simulink model "stepMotor"  (R2023b)
settings: Solver=FixedStepDiscrete  StartTime=0.0  StopTime=0.5  FixedStep=0.0001  RelTol=1e-3  EnableMultiTasking=on
undefined symbols (not defined in the file or in its folder): direction, enable, enSave, moveDown, moveRange, moveUp, steps, timeStamp, trig
libraries: simulink x12, dspswit3 x3
settings Model: DataDictionary=DD.sldd  Creator=HC  LastModifiedBy=HC
settings OptimizationCC: DefaultParameterBehavior=Inlined  EnhancedBackFolding=on  PassReuseOutputArgsAs=Individual arguments  ZeroExternalMemoryAtStartup=off  ZeroInternalMemoryAtStartup=off  MaxStackSize=64  OptimizeBlockOrder=speed  DifferentSizesBufferReuse=on  OptimizationCustomize=off  EfficientTunableParamExpr=on
settings DebuggingCC: ParameterTunabilityLossMsg=error
settings HardwareCC: ProdBitPerPointer=32  ProdBitPerSizeT=32  ProdBitPerPtrDiffT=32  ProdLargestAtomicInteger=Long  ProdLargestAtomicFloat=Double  ProdWordSize=32  ProdHWDeviceType=ARM Compatible->ARM Cortex-M
settings ModelReferenceCC: ModelReferenceNumInstancesAllowed=Single
settings SFSimCC: MATLABDynamicMemAlloc=off
settings RTWCC: Description=Embedded Coder  SystemTargetFile=ert.tlc  GenCodeOnly=on  TemplateMakefile=ert_default_tmf  Toolchain=GNU Tools for ARM Embedded Processors
settings CodeAppCC: ForceParamTrailComments=on  IgnoreCustomStorageClasses=off  OperatorAnnotations=on  SimulinkDataObjDesc=on  SFDataObjDesc=on  InsertBlockDesc=on
settings ERTTargetCC: TargetLangStandard=C99 (ISO)  InlinedParameterPlacement=NonHierarchical  ERTCustomFileTemplate=example_file_process.tlc

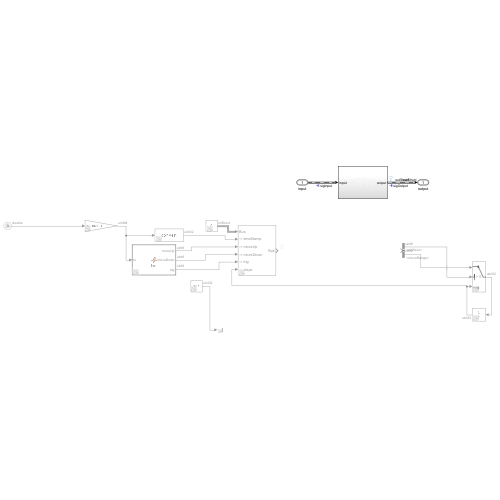
[thumbnail: Simulink's stored preview of the top-level diagram]
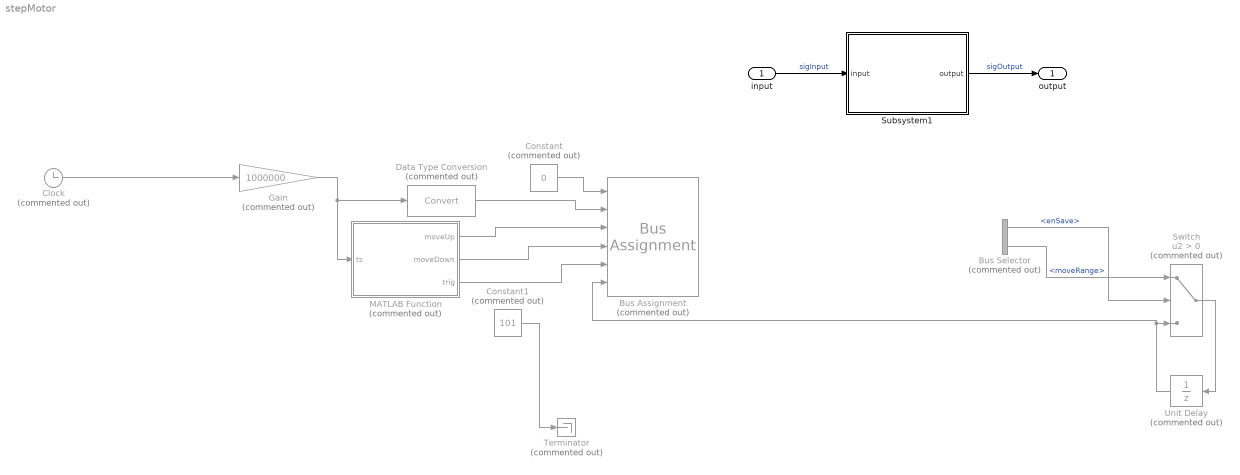
== system stepMotor ==
  input : Inport  OutDataTypeStr=Bus: inStruct
  Bus Assignment : BusAssignment  Commented=on  AssignedSignals=timeStamp,moveUp,moveDown,trig,steps
  Bus Selector : BusSelector  Commented=on  OutputSignals=enSave,moveRange
  Clock : Clock  Commented=on
  Constant : Constant  Commented=on  Value=0  OutDataTypeStr=Bus: inStruct
  Constant1 : Constant  Commented=on  Value=101  OutDataTypeStr=uint32
  Data Type Conversion : DataTypeConversion  Commented=on  SaturateOnIntegerOverflow=off  RndMeth=Floor
  Gain : Gain  Commented=on  Gain=1000000  OutDataTypeStr=uint64
  MATLAB Function : MATLAB Function  Commented=on  TreatAsAtomicUnit=on
  Subsystem1 : Subsystem
  Switch : Switch  Commented=on  Criteria=u2 > Threshold  SaturateOnIntegerOverflow=off  InputSameDT=off
  Terminator : Terminator  Commented=on
  Unit Delay : UnitDelay  Commented=on  SampleTime=-1  HasFrameUpgradeWarning=on
  output : Outport  OutDataTypeStr=Bus: outStruct
  wires:
  Subsystem1/1(output) -> output/1  "sigOutput"
  input/1 -> Subsystem1/1(input)  "sigInput"
  Constant/1 -> Bus Assignment/1
  Gain/1 -> MATLAB Function/1(ts), Data Type Conversion/1
  MATLAB Function/1(moveUp) -> Bus Assignment/3
  MATLAB Function/2(moveDown) -> Bus Assignment/4
  MATLAB Function/3(trig) -> Bus Assignment/5
  Bus Selector/1 -> Switch/2  "<enSave>"
  Bus Selector/2 -> Switch/1  "<moveRange>"
  Switch/1 -> Unit Delay/1
  Unit Delay/1 -> Bus Assignment/6, Switch/3
  Constant1/1 -> Terminator/1
  Clock/1 -> Gain/1
  Data Type Conversion/1 -> Bus Assignment/2

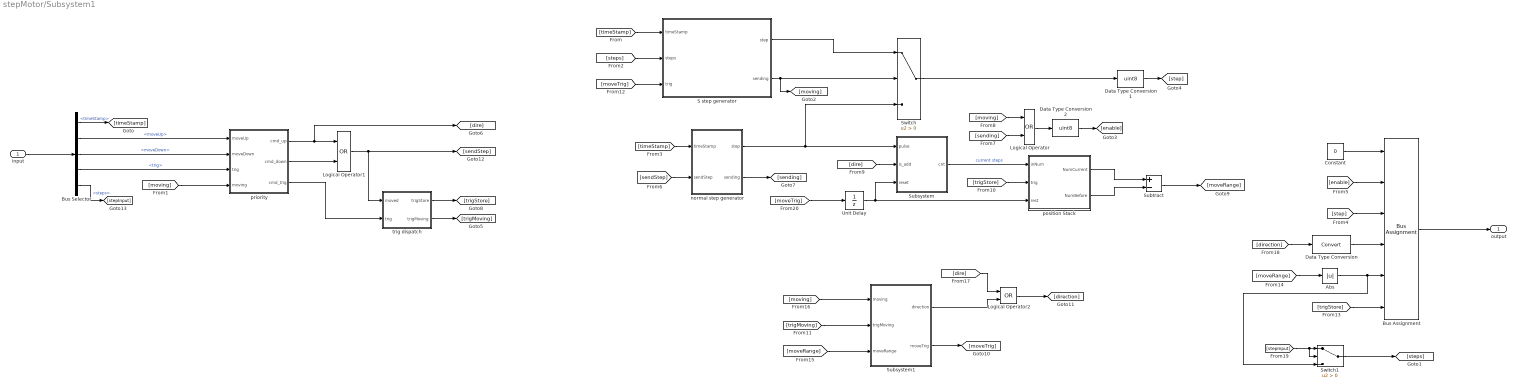
== system stepMotor/Subsystem1 ==
  input : Inport
  Abs : Abs  SaturateOnIntegerOverflow=off
  Bus Assignment : BusAssignment  AssignedSignals=enable,step,direction,moveRange,enSave
  Bus Selector : BusSelector  OutputSignals=timeStamp,moveUp,moveDown,trig,steps
  Constant : Constant  Value=0  OutDataTypeStr=Bus: outStruct
  Data Type Conversion : DataTypeConversion  SaturateOnIntegerOverflow=off  RndMeth=Floor
  Data Type Conversion1 : DataTypeConversion  OutDataTypeStr=uint8  SaturateOnIntegerOverflow=off  RndMeth=Floor
  Data Type Conversion2 : DataTypeConversion  OutDataTypeStr=uint8  SaturateOnIntegerOverflow=off  RndMeth=Floor
  Logical Operator : Logic  Operator=OR  AllPortsSameDT=off  OutDataTypeStr=boolean
  Logical Operator1 : Logic  Operator=OR  AllPortsSameDT=off  OutDataTypeStr=boolean
  Logical Operator2 : Logic  Operator=OR  AllPortsSameDT=off  OutDataTypeStr=boolean
  S step generator : Subsystem
  Subsystem : Subsystem
  Subsystem1 : Subsystem
  Subtract : Sum  Inputs=+-
  Switch : Switch  Criteria=u2 > Threshold  SaturateOnIntegerOverflow=off  InputSameDT=off
  Switch1 : Switch  Criteria=u2 > Threshold  SaturateOnIntegerOverflow=off  InputSameDT=off
  Unit Delay : UnitDelay  SampleTime=-1  HasFrameUpgradeWarning=on
  normal step generator : Subsystem
  position Stack : Subsystem
  priority : Subsystem
  trig dispatch : Subsystem
  output : Outport
  wires:
  [timeStamp] -> S step generator/1(timeStamp)
  normal step generator/1(step) -> Subsystem/1(pulse), Switch/3
  Constant/1 -> Bus Assignment/1
  Bus Assignment/1 -> output/1
  Data Type Conversion2/1 -> [enable]
  Data Type Conversion1/1 -> [step]
  [moveTrig] -> S step generator/3(trig)
  Logical Operator/1 -> Data Type Conversion2/1
  [direction] -> Data Type Conversion/1
  [timeStamp] -> normal step generator/1(timeStamp)
  S step generator/2(sending) -> [moving], Switch/2
  [step] -> Bus Assignment/3
  S step generator/1(step) -> Switch/1
  [steps] -> S step generator/2(steps)
  [enable] -> Bus Assignment/2
  Switch/1 -> Data Type Conversion1/1
  normal step generator/2(sending) -> [sending]
  input/1 -> Bus Selector/1
  Bus Selector/1 -> [timeStamp]  "<timeStamp>"
  Bus Selector/2 -> priority/1(moveUp)  "<moveUp>"
  Bus Selector/4 -> priority/3(trig)  "<trig>"
  Bus Selector/5 -> [stepInput]  "<steps>"
  trig dispatch/2(trigMoving) -> [trigMoving]
  priority/1(cmd_up) -> [dire], Logical Operator1/1
  Bus Selector/3 -> priority/2(moveDown)  "<moveDown>"
  priority/2(cmd_down) -> Logical Operator1/2
  Subsystem/1(cnt) -> position Stack/1(inNum)  "current steps"
  [moving] -> Logical Operator/1
  [sending] -> Logical Operator/2
  [dire] -> Subsystem/2(is_add)
  Data Type Conversion/1 -> Bus Assignment/4
  Unit Delay/1 -> Subsystem/3(reset), position Stack/3(rest)
  Logical Operator1/1 -> [sendStep], trig dispatch/1(moved)
  priority/3(cmd_trig) -> trig dispatch/2(trig)
  [moving] -> priority/4(moving)
  trig dispatch/1(trigStore) -> [trigStore]
  [trigStore] -> position Stack/2(trig)
  position Stack/1(NumCurrent) -> Subtract/1
  position Stack/2(NumBefore) -> Subtract/2
  [moveRange] -> Abs/1
  Subtract/1 -> [moveRange]
  [trigStore] -> Bus Assignment/6
  Abs/1 -> Switch1/3, Bus Assignment/5
  [moving] -> Subsystem1/1(moving)
  [trigMoving] -> Subsystem1/2(trigMoving)
  [moveRange] -> Subsystem1/3(moveRange)
  Subsystem1/1(direction) -> Logical Operator2/2
  Subsystem1/2(moveTrig) -> [moveTrig]
  [dire] -> Logical Operator2/1
  Logical Operator2/1 -> [direction]
  [sendStep] -> normal step generator/2(sendStep)
  [stepInput] -> Switch1/2, Switch1/1
  Switch1/1 -> [steps]
  [moveTrig] -> Unit Delay/1

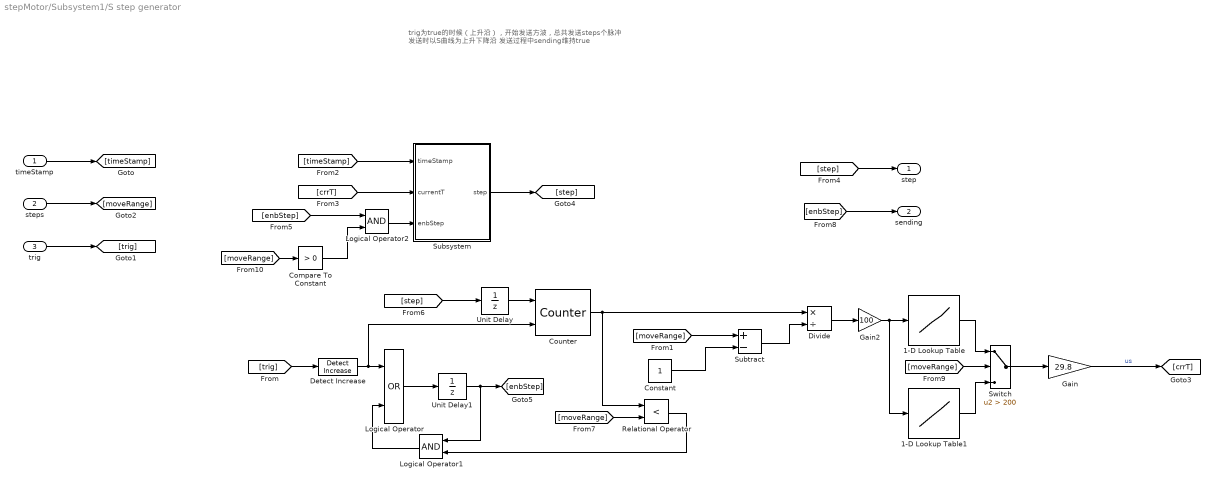
== system stepMotor/Subsystem1/S step generator ==
  note: trig为true的时候（上升沿），开始发送方波，总共发送steps个脉冲
      | 发送时以S曲线为上升下降沿
      | 发送过程中sending维持true
  timeStamp : Inport
  steps : Inport  Port=2
  trig : Inport  Port=3
  1-D Lookup Table : Lookup_n-D  NumberOfTableDimensions=1  BreakpointsForDimension1=[0;1;2;3;4;5;6;94;95;96;97;98;99;100]  Table=[10.0250134994341;4.32011692273655;2.22140275816017;1.44932896411722;1.16529888822159;1.06081006262522;1.02237077185617;1.02237077185617;1.06081006262522;1.16529888822159;1.44932896411722;2.22140275816017;4.32011692273655;10.0250134994341]  ExtrapMethod=Clip  UseLastTableValue=on  InternalRulePriority=Speed  RndMeth=Simplest
  1-D Lookup Table1 : Lookup_n-D  NumberOfTableDimensions=1  BreakpointsForDimension1=[0;1;3;6;10;16;25;74;85;91;95;98;99;100]  Table=[10;9.1;7.6;5.8;4;2.3;1;1;2.3;4;5.8;7.6;9.1;10]  ExtrapMethod=Clip  UseLastTableValue=on  InternalRulePriority=Speed  RndMeth=Simplest
  Compare To Constant : simulink/Logic and Bit Operations/Compare To Constant  relop=>  const=0  OutDataTypeStr=boolean
  Constant : Constant
  Counter : dspswit3/Counter  Direction=Up  CountEvent=Falling edge  CounterSize=32 bits  MaxCount=255  InitialCount=0  Output=Count  HitValue=32  ResetInput=on  SamplesPerFrame=1  Ts=1  CntDtype=uint32  HitDtype=Logical
  Detect Increase : simulink/Logic and Bit Operations/Detect Increase  vinit=0.0  OutDataTypeStr=boolean
  Divide : Product  Inputs=*/  OutDataTypeStr=single
  Gain : Gain  Gain=29.8
  Gain2 : Gain  Gain=100
  Logical Operator : Logic  Operator=OR  AllPortsSameDT=off  OutDataTypeStr=boolean
  Logical Operator1 : Logic  AllPortsSameDT=off  OutDataTypeStr=boolean
  Logical Operator2 : Logic  AllPortsSameDT=off  OutDataTypeStr=boolean
  Relational Operator : RelationalOperator  Operator=<  OutDataTypeStr=boolean  RndMeth=Simplest  InputSameDT=off
  Subsystem : Subsystem
  Subtract : Sum  Inputs=+-
  Switch : Switch  Criteria=u2 > Threshold  Threshold=200  SaturateOnIntegerOverflow=off  InputSameDT=off
  Unit Delay : UnitDelay  SampleTime=-1  HasFrameUpgradeWarning=on
  Unit Delay1 : UnitDelay  SampleTime=-1  HasFrameUpgradeWarning=on
  step : Outport
  sending : Outport  Port=2
  wires:
  [moveRange] -> Relational Operator/2
  Detect Increase/1 -> Counter/2, Logical Operator/1
  Subsystem/1(step) -> [step]
  Counter/1 -> Relational Operator/1, Divide/1
  Logical Operator1/1 -> Logical Operator/2
  [trig] -> Detect Increase/1
  Logical Operator/1 -> Unit Delay1/1
  Divide/1 -> Gain2/1
  [crrT] -> Subsystem/2(currentT)
  [moveRange] -> Subtract/1
  Gain2/1 -> 1-D Lookup Table1/1, 1-D Lookup Table/1
  1-D Lookup Table/1 -> Switch/1
  Relational Operator/1 -> Logical Operator1/2
  [step] -> Unit Delay/1
  Unit Delay/1 -> Counter/1
  Gain/1 -> [crrT]  "us"
  [timeStamp] -> Subsystem/1(timeStamp)
  Unit Delay1/1 -> [enbStep], Logical Operator1/1
  [step] -> step/1
  timeStamp/1 -> [timeStamp]
  steps/1 -> [moveRange]
  trig/1 -> [trig]
  [enbStep] -> sending/1
  Logical Operator2/1 -> Subsystem/3(enbStep)
  Subtract/1 -> Divide/2
  Constant/1 -> Subtract/2
  Switch/1 -> Gain/1
  1-D Lookup Table1/1 -> Switch/3
  [moveRange] -> Switch/2
  [moveRange] -> Compare To Constant/1
  Compare To Constant/1 -> Logical Operator2/2
  [enbStep] -> Logical Operator2/1

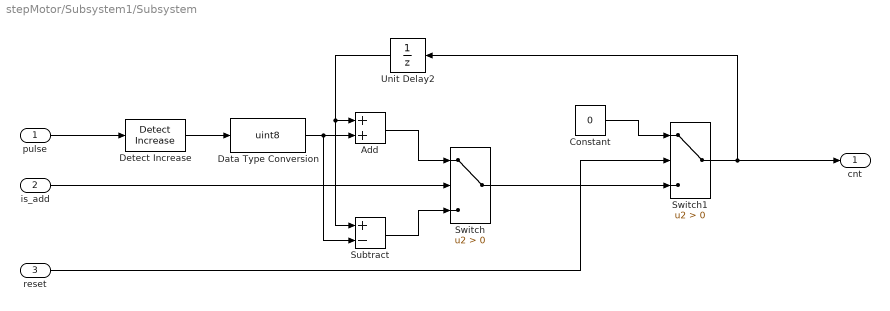
== system stepMotor/Subsystem1/Subsystem ==
  pulse : Inport
  is_add : Inport  Port=2
  reset : Inport  Port=3
  Add : Sum
  Constant : Constant  Value=0  OutDataTypeStr=int32
  Data Type Conversion : DataTypeConversion  OutDataTypeStr=uint8  SaturateOnIntegerOverflow=off  RndMeth=Floor
  Detect Increase : simulink/Logic and Bit Operations/Detect Increase  vinit=0.0  OutDataTypeStr=boolean
  Subtract : Sum  Inputs=+-
  Switch : Switch  Criteria=u2 > Threshold  SaturateOnIntegerOverflow=off  InputSameDT=off
  Switch1 : Switch  Criteria=u2 > Threshold  OutDataTypeStr=int32  SaturateOnIntegerOverflow=off  InputSameDT=off
  Unit Delay2 : UnitDelay  SampleTime=-1  HasFrameUpgradeWarning=on
  cnt : Outport
  wires:
  Unit Delay2/1 -> Add/1, Subtract/1
  is_add/1 -> Switch/2
  Data Type Conversion/1 -> Subtract/2, Add/2
  Switch/1 -> Switch1/3
  Detect Increase/1 -> Data Type Conversion/1
  Switch1/1 -> Unit Delay2/1, cnt/1
  Add/1 -> Switch/1
  Subtract/1 -> Switch/3
  pulse/1 -> Detect Increase/1
  Constant/1 -> Switch1/1
  reset/1 -> Switch1/2

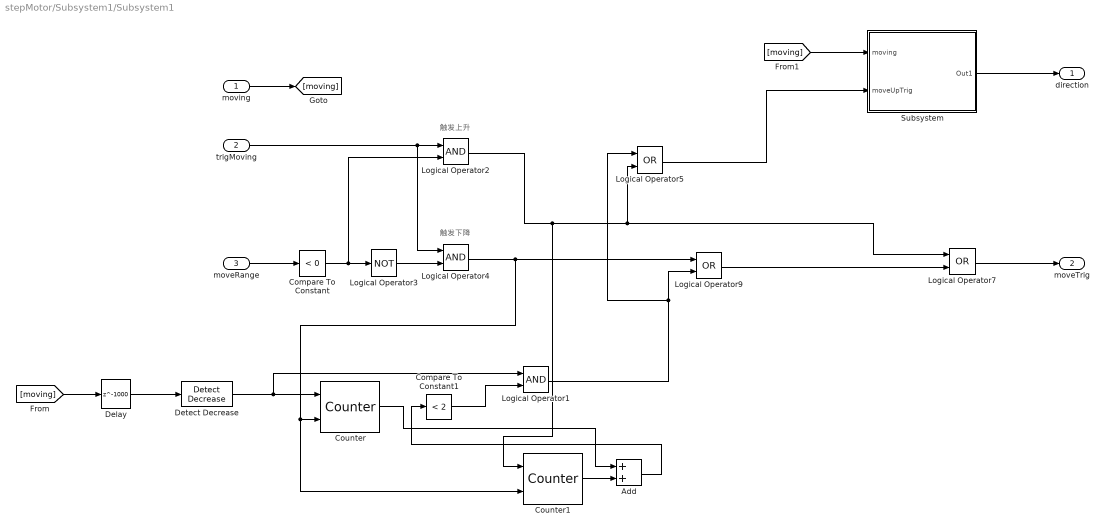
== system stepMotor/Subsystem1/Subsystem1 ==
  note: 触发下降
  note: 触发上升
  moving : Inport
  trigMoving : Inport  Port=2
  moveRange : Inport  Port=3
  Add : Sum
  Compare To Constant : simulink/Logic and Bit Operations/Compare To Constant  relop=<  const=0  OutDataTypeStr=boolean
  Compare To Constant1 : simulink/Logic and Bit Operations/Compare To Constant  relop=<  const=2  OutDataTypeStr=boolean
  Counter : dspswit3/Counter  Direction=Up  CountEvent=Rising edge  CounterSize=8 bits  MaxCount=255  InitialCount=0  Output=Count  HitValue=32  ResetInput=on  SamplesPerFrame=1  Ts=1  CntDtype=uint8  HitDtype=Logical
  Counter1 : dspswit3/Counter  Direction=Up  CountEvent=Rising edge  CounterSize=8 bits  MaxCount=255  InitialCount=0  Output=Count  HitValue=32  ResetInput=on  SamplesPerFrame=1  Ts=1  CntDtype=uint8  HitDtype=Logical
  Delay : Delay  DelayLength=1000
  Detect Decrease : simulink/Logic and Bit Operations/Detect Decrease  vinit=0.0  OutDataTypeStr=boolean
  Logical Operator1 : Logic  AllPortsSameDT=off  OutDataTypeStr=boolean
  Logical Operator2 : Logic  AllPortsSameDT=off  OutDataTypeStr=boolean
  Logical Operator3 : Logic  Operator=NOT  AllPortsSameDT=off  OutDataTypeStr=boolean
  Logical Operator4 : Logic  AllPortsSameDT=off  OutDataTypeStr=boolean
  Logical Operator5 : Logic  Operator=OR  AllPortsSameDT=off  OutDataTypeStr=boolean
  Logical Operator7 : Logic  Operator=OR  AllPortsSameDT=off  OutDataTypeStr=boolean
  Logical Operator9 : Logic  Operator=OR  AllPortsSameDT=off  OutDataTypeStr=boolean
  Subsystem : Subsystem
  direction : Outport
  moveTrig : Outport  Port=2
  wires:
  trigMoving/1 -> Logical Operator4/1, Logical Operator2/1
  Logical Operator2/1 -> Counter1/1, Logical Operator5/2, Logical Operator7/1
  Compare To Constant/1 -> Logical Operator3/1, Logical Operator2/2
  Logical Operator3/1 -> Logical Operator4/2
  moving/1 -> [moving]
  moveRange/1 -> Compare To Constant/1
  [moving] -> Delay/1
  Logical Operator7/1 -> moveTrig/1
  Logical Operator9/1 -> Logical Operator7/2
  Delay/1 -> Detect Decrease/1
  Logical Operator4/1 -> Counter1/2, Counter/2, Logical Operator9/1
  [moving] -> Subsystem/1(moving)
  Subsystem/1(Out1) -> direction/1
  Compare To Constant1/1 -> Logical Operator1/2
  Detect Decrease/1 -> Logical Operator1/1, Counter/1
  Counter/1 -> Add/1
  Logical Operator1/1 -> Logical Operator5/1, Logical Operator9/2
  Logical Operator5/1 -> Subsystem/2(moveUpTrig)
  Counter1/1 -> Add/2
  Add/1 -> Compare To Constant1/1

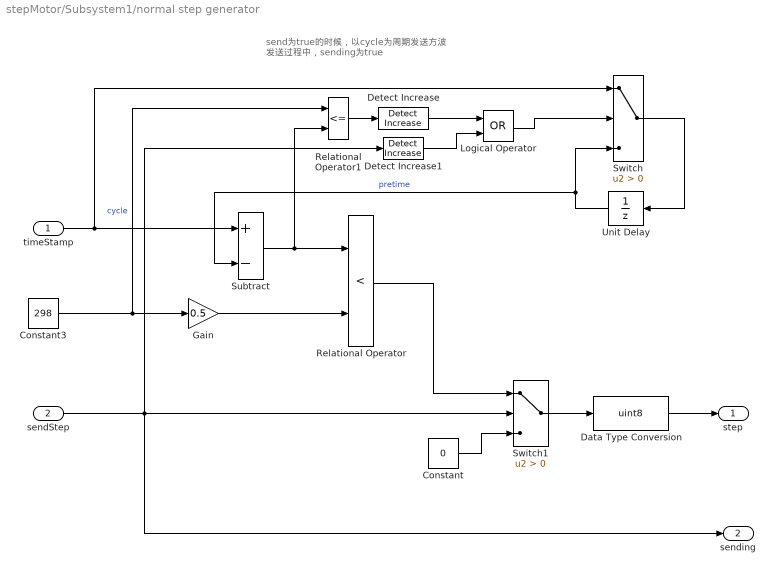
== system stepMotor/Subsystem1/normal step generator ==
  note: send为true的时候，以cycle为周期发送方波
      | 发送过程中，sending为true
  timeStamp : Inport
  sendStep : Inport  Port=2
  Constant : Constant  Value=0  OutDataTypeStr=boolean
  Constant3 : Constant  Value=298
  Data Type Conversion : DataTypeConversion  OutDataTypeStr=uint8  SaturateOnIntegerOverflow=off  RndMeth=Floor
  Detect Increase : simulink/Logic and Bit Operations/Detect Increase  vinit=0.0  OutDataTypeStr=boolean
  Detect Increase1 : simulink/Logic and Bit Operations/Detect Increase  vinit=0.0  OutDataTypeStr=boolean
  Gain : Gain  Gain=0.5
  Logical Operator : Logic  Operator=OR  AllPortsSameDT=off  OutDataTypeStr=boolean
  Relational Operator : RelationalOperator  Operator=<  OutDataTypeStr=boolean  RndMeth=Simplest  InputSameDT=off
  Relational Operator1 : RelationalOperator  Operator=<=  OutDataTypeStr=boolean  RndMeth=Simplest  InputSameDT=off
  Subtract : Sum  Inputs=+-
  Switch : Switch  Criteria=u2 > Threshold  SaturateOnIntegerOverflow=off  InputSameDT=off
  Switch1 : Switch  Criteria=u2 > Threshold  SaturateOnIntegerOverflow=off  InputSameDT=off
  Unit Delay : UnitDelay  SampleTime=-1  HasFrameUpgradeWarning=on
  step : Outport
  sending : Outport  Port=2
  wires:
  Unit Delay/1 -> Subtract/2, Switch/3  "pretime"
  Switch/1 -> Unit Delay/1
  Relational Operator/1 -> Switch1/1
  Detect Increase/1 -> Logical Operator/1
  Subtract/1 -> Relational Operator1/2, Relational Operator/1
  timeStamp/1 -> Subtract/1, Switch/1
  Gain/1 -> Relational Operator/2
  Constant3/1 -> Relational Operator1/1, Gain/1  "cycle"
  Relational Operator1/1 -> Detect Increase/1
  sendStep/1 -> sending/1, Detect Increase1/1, Switch1/2
  Switch1/1 -> Data Type Conversion/1
  Constant/1 -> Switch1/3
  Data Type Conversion/1 -> step/1
  Detect Increase1/1 -> Logical Operator/2
  Logical Operator/1 -> Switch/2

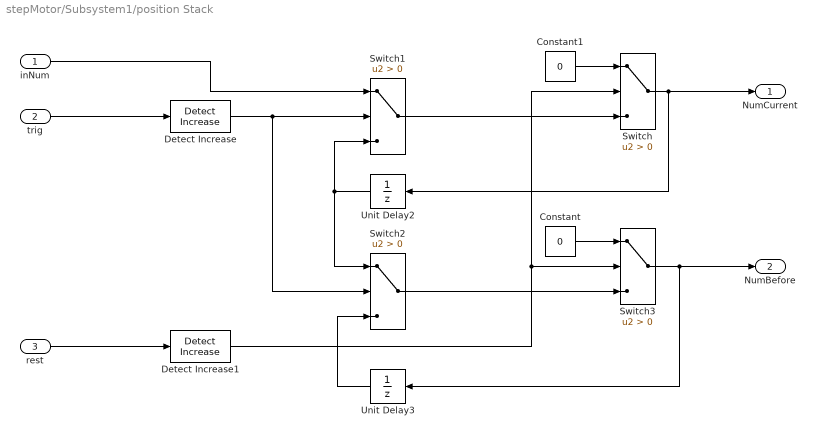
== system stepMotor/Subsystem1/position Stack ==
  inNum : Inport
  trig : Inport  Port=2
  rest : Inport  Port=3
  Constant : Constant  Value=0  OutDataTypeStr=int32
  Constant1 : Constant  Value=0  OutDataTypeStr=int32
  Detect Increase : simulink/Logic and Bit Operations/Detect Increase  vinit=0.0  OutDataTypeStr=boolean
  Detect Increase1 : simulink/Logic and Bit Operations/Detect Increase  vinit=0.0  OutDataTypeStr=boolean
  Switch{,1..3} (4 alike) : Switch  Criteria=u2 > Threshold  SaturateOnIntegerOverflow=off  InputSameDT=off
  Unit Delay2 : UnitDelay  SampleTime=-1  HasFrameUpgradeWarning=on
  Unit Delay3 : UnitDelay  SampleTime=-1  HasFrameUpgradeWarning=on
  NumCurrent : Outport
  NumBefore : Outport  Port=2
  wires:
  Switch1/1 -> Switch/3
  Unit Delay3/1 -> Switch2/3
  inNum/1 -> Switch1/1
  Switch2/1 -> Switch3/3
  Unit Delay2/1 -> Switch2/1, Switch1/3
  Detect Increase/1 -> Switch2/2, Switch1/2
  trig/1 -> Detect Increase/1
  Switch/1 -> NumCurrent/1, Unit Delay2/1
  Switch3/1 -> Unit Delay3/1, NumBefore/1
  Constant/1 -> Switch3/1
  Constant1/1 -> Switch/1
  Detect Increase1/1 -> Switch3/2, Switch/2
  rest/1 -> Detect Increase1/1

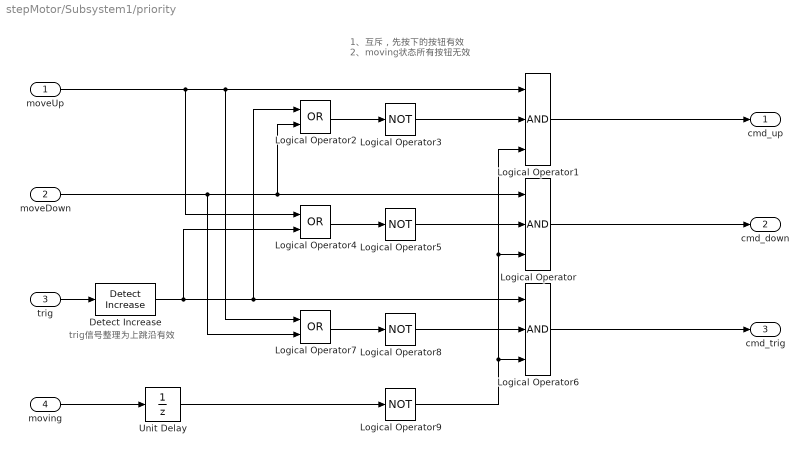
== system stepMotor/Subsystem1/priority ==
  note: trig信号整理为上跳沿有效
  note: 1、互斥，先按下的按钮有效
      | 2、moving状态所有按钮无效
  moveUp : Inport
  moveDown : Inport  Port=2
  trig : Inport  Port=3
  moving : Inport  Port=4
  Detect Increase : simulink/Logic and Bit Operations/Detect Increase  vinit=0.0  OutDataTypeStr=boolean
  Logical Operator : Logic  Inputs=3  AllPortsSameDT=off  OutDataTypeStr=boolean
  Logical Operator1 : Logic  Inputs=3  AllPortsSameDT=off  OutDataTypeStr=boolean
  Logical Operator2 : Logic  Operator=OR  AllPortsSameDT=off  OutDataTypeStr=boolean
  Logical Operator{3,5,8..9} (4 alike) : Logic  Operator=NOT  AllPortsSameDT=off  OutDataTypeStr=boolean
  Logical Operator4 : Logic  Operator=OR  AllPortsSameDT=off  OutDataTypeStr=boolean
  Logical Operator6 : Logic  Inputs=3  AllPortsSameDT=off  OutDataTypeStr=boolean
  Logical Operator7 : Logic  Operator=OR  AllPortsSameDT=off  OutDataTypeStr=boolean
  Unit Delay : UnitDelay  SampleTime=-1  HasFrameUpgradeWarning=on
  cmd_up : Outport
  cmd_down : Outport  Port=2
  cmd_trig : Outport  Port=3
  wires:
  moveUp/1 -> Logical Operator4/1, Logical Operator7/1, Logical Operator1/1
  Logical Operator/1 -> cmd_down/1
  moveDown/1 -> Logical Operator7/2, Logical Operator2/2, Logical Operator/1
  Logical Operator4/1 -> Logical Operator5/1
  Logical Operator3/1 -> Logical Operator1/2
  Logical Operator6/1 -> cmd_trig/1
  Logical Operator1/1 -> cmd_up/1
  Detect Increase/1 -> Logical Operator4/2, Logical Operator2/1, Logical Operator6/1
  Logical Operator2/1 -> Logical Operator3/1
  Logical Operator7/1 -> Logical Operator8/1
  Logical Operator5/1 -> Logical Operator/2
  Logical Operator8/1 -> Logical Operator6/2
  moving/1 -> Unit Delay/1
  Logical Operator9/1 -> Logical Operator1/3, Logical Operator/3, Logical Operator6/3
  Unit Delay/1 -> Logical Operator9/1
  trig/1 -> Detect Increase/1

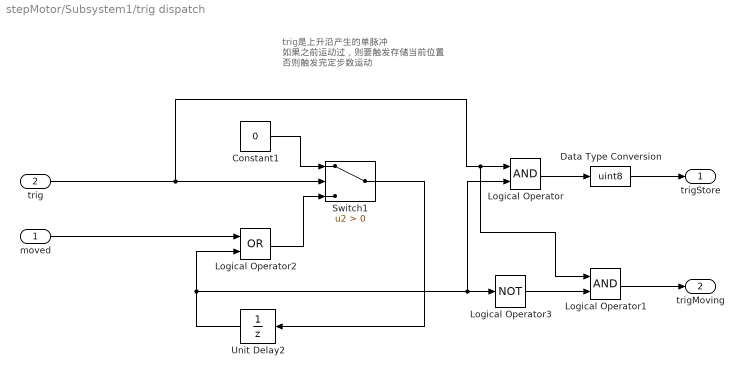
== system stepMotor/Subsystem1/trig dispatch ==
  note: trig是上升沿产生的单脉冲
      | 如果之前运动过，则要触发存储当前位置
      | 否则触发完定步数运动
  moved : Inport
  trig : Inport  Port=2
  Constant1 : Constant  Value=0  OutDataTypeStr=boolean
  Data Type Conversion : DataTypeConversion  OutDataTypeStr=uint8  SaturateOnIntegerOverflow=off  RndMeth=Floor
  Logical Operator : Logic  AllPortsSameDT=off  OutDataTypeStr=boolean
  Logical Operator1 : Logic  AllPortsSameDT=off  OutDataTypeStr=boolean
  Logical Operator2 : Logic  Operator=OR  AllPortsSameDT=off  OutDataTypeStr=boolean
  Logical Operator3 : Logic  Operator=NOT  AllPortsSameDT=off  OutDataTypeStr=boolean
  Switch1 : Switch  Criteria=u2 > Threshold  SaturateOnIntegerOverflow=off  InputSameDT=off
  Unit Delay2 : UnitDelay  SampleTime=-1  HasFrameUpgradeWarning=on
  trigStore : Outport
  trigMoving : Outport  Port=2
  wires:
  Logical Operator2/1 -> Switch1/3
  trig/1 -> Logical Operator1/1, Logical Operator/1, Switch1/2
  Constant1/1 -> Switch1/1
  Switch1/1 -> Unit Delay2/1
  moved/1 -> Logical Operator2/1
  Unit Delay2/1 -> Logical Operator2/2, Logical Operator/2, Logical Operator3/1
  Logical Operator/1 -> Data Type Conversion/1
  Logical Operator3/1 -> Logical Operator1/2
  Logical Operator1/1 -> trigMoving/1
  Data Type Conversion/1 -> trigStore/1

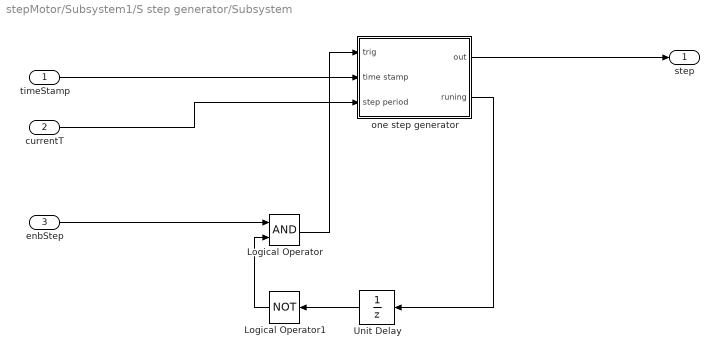
== system stepMotor/Subsystem1/S step generator/Subsystem ==
  timeStamp : Inport
  currentT : Inport  Port=2
  enbStep : Inport  Port=3
  Logical Operator : Logic  AllPortsSameDT=off  OutDataTypeStr=boolean
  Logical Operator1 : Logic  Operator=NOT  AllPortsSameDT=off  OutDataTypeStr=boolean
  Unit Delay : UnitDelay  SampleTime=-1  HasFrameUpgradeWarning=on
  one step generator : Subsystem
  step : Outport
  wires:
  timeStamp/1 -> one step generator/2(time stamp)
  currentT/1 -> one step generator/3(step period)
  enbStep/1 -> Logical Operator/1
  one step generator/1(out) -> step/1
  Logical Operator1/1 -> Logical Operator/2
  one step generator/2(runing) -> Unit Delay/1
  Logical Operator/1 -> one step generator/1(trig)
  Unit Delay/1 -> Logical Operator1/1

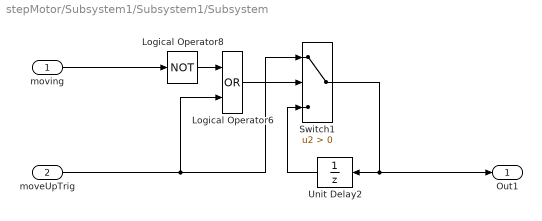
== system stepMotor/Subsystem1/Subsystem1/Subsystem ==
  moving : Inport
  moveUpTrig : Inport  Port=2
  Logical Operator6 : Logic  Operator=OR  AllPortsSameDT=off  OutDataTypeStr=boolean
  Logical Operator8 : Logic  Operator=NOT  AllPortsSameDT=off  OutDataTypeStr=boolean
  Switch1 : Switch  Criteria=u2 > Threshold  SaturateOnIntegerOverflow=off  InputSameDT=off
  Unit Delay2 : UnitDelay  SampleTime=-1  HasFrameUpgradeWarning=on
  Out1 : Outport
  wires:
  Logical Operator8/1 -> Logical Operator6/1
  moveUpTrig/1 -> Switch1/1, Logical Operator6/2
  Unit Delay2/1 -> Switch1/3
  Switch1/1 -> Out1/1, Unit Delay2/1
  Logical Operator6/1 -> Switch1/2
  moving/1 -> Logical Operator8/1

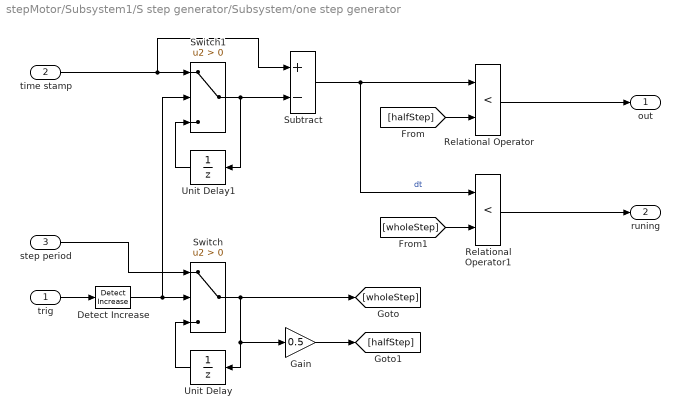
== system stepMotor/Subsystem1/S step generator/Subsystem/one step generator ==
  trig : Inport
  time stamp : Inport  Port=2
  step period : Inport  Port=3
  Detect Increase : simulink/Logic and Bit Operations/Detect Increase  vinit=0.0  OutDataTypeStr=boolean
  Gain : Gain  Gain=0.5
  Relational Operator : RelationalOperator  Operator=<  OutDataTypeStr=boolean  RndMeth=Simplest  InputSameDT=off
  Relational Operator1 : RelationalOperator  Operator=<  OutDataTypeStr=boolean  RndMeth=Simplest  InputSameDT=off
  Subtract : Sum  Inputs=+-
  Switch : Switch  Criteria=u2 > Threshold  SaturateOnIntegerOverflow=off  InputSameDT=off
  Switch1 : Switch  Criteria=u2 > Threshold  SaturateOnIntegerOverflow=off  InputSameDT=off
  Unit Delay : UnitDelay  SampleTime=-1  HasFrameUpgradeWarning=on
  Unit Delay1 : UnitDelay  SampleTime=-1  HasFrameUpgradeWarning=on
  out : Outport
  runing : Outport  Port=2
  wires:
  trig/1 -> Detect Increase/1
  Switch/1 -> Gain/1, Unit Delay/1, [wholeStep]
  Gain/1 -> [halfStep]
  Unit Delay/1 -> Switch/3
  step period/1 -> Switch/1
  Detect Increase/1 -> Switch1/2, Switch/2
  Unit Delay1/1 -> Switch1/3
  Switch1/1 -> Subtract/2, Unit Delay1/1
  time stamp/1 -> Subtract/1, Switch1/1
  Subtract/1 -> Relational Operator1/1, Relational Operator/1  "dt"
  [halfStep] -> Relational Operator/2
  Relational Operator/1 -> out/1
  [wholeStep] -> Relational Operator1/2
  Relational Operator1/1 -> runing/1

== matlab function stepMotor/MATLAB Function ==
  data: ts input uint64; moveUp output uint8; moveDown output uint8; trig output uint8
function [moveUp, moveDown, trig] = fcn(ts)
    moveUp = uint8(0);
    moveDown = uint8(0);
    trig = uint8(0);

    if(ts>100000 && ts <200000) % 0.1s-0.2s
        moveDown = uint8(1);
    end

    if(ts>280000 && ts <290000) % 0.28s-0.29s
        trig = uint8(1);
    end

    if(ts>300000 && ts <350000) % 0.30s-0.35s
        moveUp = uint8(1);
    end

    if(ts>360000 && ts <370000) % 0.36s-0.37s
        trig = uint8(1);
    end

    if(ts>380000 && ts <390000) % 0.38s-0.39s
        trig = uint8(1);
    end

    if(ts>400000 && ts <410000) % 0.4s-0.41s
        trig = uint8(1);
    end

    if(ts>420000 && ts <430000) % 0.42s-0.43s
        trig = uint8(1);
    end
end
